simulink model "rob_dynModel"  (R2022b)
settings: Solver=VariableStepAuto  StartTime=0.0  StopTime=100  RelTol=1e-3
values from neighbouring files (symbols this model uses):
  B1 = 2    [inputConstants.m]    (also in inputContants.mat)
  B2 = 2    [inputConstants.m]    (also in inputContants.mat)
  g = 9.81    [inputConstants.m]    (also in inputContants.mat)
  l1 = 0.75    [inputConstants.m]    (also in inputContants.mat)
  l2 = 0.75    [inputConstants.m]    (also in inputContants.mat)
  m1 = 10    [inputConstants.m]    (also in inputContants.mat)
  m2 = 10    [inputConstants.m]    (also in inputContants.mat)
undefined symbols (not defined in the file or in its folder): sigbuilder_block
libraries: simulink_extras x4, slpidlib x2
settings Model: Creator=Marek Sýkorka  LastModifiedBy=Marek Sýkorka

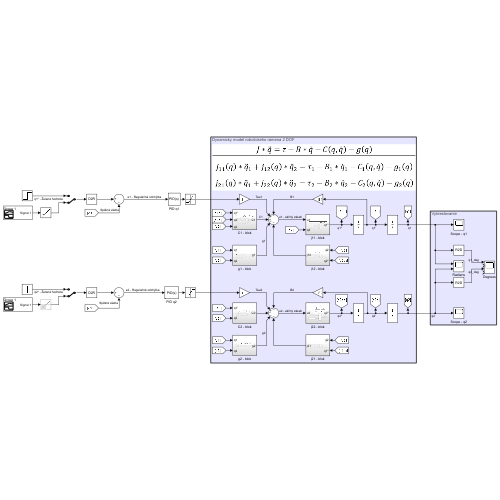
[thumbnail: Simulink's stored preview of the top-level diagram]
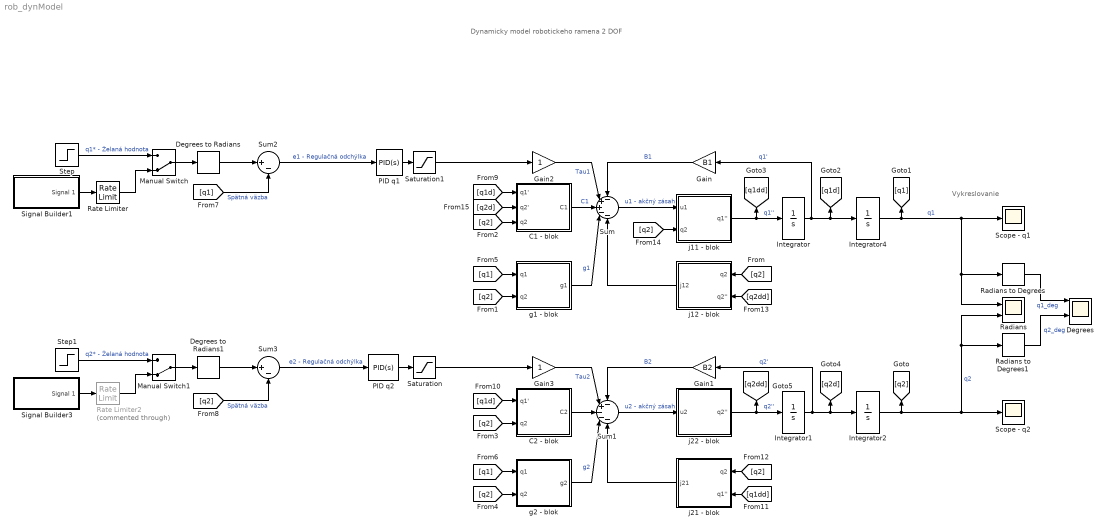
== system rob_dynModel ==
  note: Vykreslovanie
  note: Dynamicky model robotickeho ramena 2 DOF
  C1 - blok : Subsystem
  C2 - blok : Subsystem
  Degrees : Scope  NumInputPorts=4
  Degrees to Radians : simulink_extras/Transformations/Degrees to Radians
  Degrees to Radians1 : simulink_extras/Transformations/Degrees to Radians
  Gain : Gain  Gain=B1
  Gain1 : Gain  Gain=B2
  Gain2 : Gain
  Gain3 : Gain
  Integrator{,1..2,4} (4 alike) : Integrator
  Manual Switch : ManualSwitch  CurrentSetting=0
  Manual Switch1 : ManualSwitch  CurrentSetting=0
  PID q1 : slpidlib/PID Controller  Controller=PID  Form=Parallel  TimeDomain=Continuous-time  UseExternalTs=off  SampleTime=-1  IntegratorMethod=Forward Euler  FilterMethod=Forward Euler  ControllerParametersSource=internal  P=15000  I=6500  UseKiTs=off  D=6000  N=1000  UseFilter=on  TunerSelectOption=Transfer Function Based (PID Tuner App)  ZeroCross=off  InitialConditionSource=internal  InitialConditionForIntegrator=0  InitialConditionForFilter=0  DifferentiatorICPrevScaledInput=0  ExternalReset=none  TrackingMode=off  Kt=1  LimitOutput=off  SatLimitsSource=internal  UpperSaturationLimit=inf  LowerSaturationLimit=-inf  LinearizeAsGain=on  AntiWindupMode=none  Kb=1  LimitIntegrator=off  UpperIntegratorSaturationLimit=inf  LowerIntegratorSaturationLimit=-inf  POutMin=[]  POutMax=[]  IOutMin=[]  IOutMax=[]  DOutMin=[]  DOutMax=[]  NOutMin=[]  NOutMax=[]  SumOutMin=[]  SumOutMax=[]  SaturationOutMin=[]  SaturationOutMax=[]  PParamMin=[]  PParamMax=[]  IParamMin=[]  IParamMax=[]  DParamMin=[]  DParamMax=[]  NParamMin=[]  NParamMax=[]  KbParamMin=[]  KbParamMax=[]  KtParamMin=[]  KtParamMax=[]  KbOutMin=[]  KbOutMax=[]  KtOutMin=[]  KtOutMax=[]  IntegratorOutMin=[]  IntegratorOutMax=[]  FilterOutMin=[]  FilterOutMax=[]  SumI1OutMin=[]  SumI1OutMax=[]  SumI2OutMin=[]  SumI2OutMax=[]  SumI3OutMin=[]  SumI3OutMax=[]  SumI4OutMin=[]  SumI4OutMax=[]  SumDOutMin=[]  SumDOutMax=[]  DifferentiatorOutMin=[]  DifferentiatorOutMax=[]  FilterDiffOutCoefMin=[]  FilterDiffOutCoefMax=[]  ReciprocalOutMin=[]  ReciprocalOutMax=[]  SumDenOutMin=[]  SumDenOutMax=[]  SumNumOutMin=[]  SumNumOutMax=[]  DivideOutMin=[]  DivideOutMax=[]  UdiffTsProdOutMin=[]  UdiffTsProdOutMax=[]  NTsProdOutMin=[]  NTsProdOutMax=[]  UintegralTsProdOutMin=[]  UintegralTsProdOutMax=[]  UngainTsProdOutMin=[]  UngainTsProdOutMax=[]  ClampingZeroOutDataTypeStr=Inherit: Inherit via back propagation  ClampingZeroOutMin=[]  ClampingZeroOutMax=[]  FilterDenConstantOutDataTypeStr=Inherit: Inherit via back propagation  FilterDenConstantOutMin=[]  FilterDenConstantOutMax=[]  PCopyOutDataTypeStr=Inherit: Inherit via back propagation  PCopyOutMin=[]  PCopyOutMax=[]  NCopyOutDataTypeStr=Inherit: Inherit via back propagation  NCopyOutMin=[]  NCopyOutMax=[]  IntegratorContinuousStateAttributes=''  IntegratorStateMustResolveToSignalObject=off  IntegratorRTWStateStorageClass=Auto  FilterContinuousStateAttributes=''  FilterStateMustResolveToSignalObject=off  FilterRTWStateStorageClass=Auto  ParallelPVariant=InternalParameters  IdealPVariant=Disabled  IVariant=InternalParameters  DVariant=InternalParameters  IntegratorVariant=Continuous  SatVariant=Disabled  AWVariant=Passthrough  PCopyVariant=Disabled  TRVariant=Disabled  FdbkBlocksVariant=Forward  IdealPFdbkVariant=Disabled  SatFdbkVariant=Disabled  DerivativeFilterVariant=ContFilter  NVariant=InternalParameters  NCopyVariant=Disabled  FilterICVariant=InternalICsFilter  IntegratorICVariant=InternalICs  ExternalResetVariant=Disabled  TRSumVariant=Passthrough  SumFdbkVariant=Disabled  SumVariant=Sum_PID  TsampFilterVariant=InternalTs  TsampNgainVariant=Passthrough  TsampIntegralVariant=Passthrough  ExternalSaturationOutDataTypeStr=Inherit: Same as second input
  PID q2 : slpidlib/PID Controller  Controller=PID  Form=Parallel  TimeDomain=Continuous-time  UseExternalTs=off  SampleTime=-1  IntegratorMethod=Forward Euler  FilterMethod=Forward Euler  ControllerParametersSource=internal  P=10000  I=5000  UseKiTs=off  D=4000  N=350  UseFilter=on  TunerSelectOption=Transfer Function Based (PID Tuner App)  InitialConditionSource=internal  InitialConditionForIntegrator=0  InitialConditionForFilter=0  DifferentiatorICPrevScaledInput=0  ExternalReset=none  TrackingMode=off  Kt=1  LimitOutput=off  SatLimitsSource=internal  UpperSaturationLimit=inf  LowerSaturationLimit=-inf  LinearizeAsGain=on  AntiWindupMode=none  Kb=1  LimitIntegrator=off  UpperIntegratorSaturationLimit=inf  LowerIntegratorSaturationLimit=-inf  POutMin=[]  POutMax=[]  IOutMin=[]  IOutMax=[]  DOutMin=[]  DOutMax=[]  NOutMin=[]  NOutMax=[]  SumOutMin=[]  SumOutMax=[]  SaturationOutMin=[]  SaturationOutMax=[]  PParamMin=[]  PParamMax=[]  IParamMin=[]  IParamMax=[]  DParamMin=[]  DParamMax=[]  NParamMin=[]  NParamMax=[]  KbParamMin=[]  KbParamMax=[]  KtParamMin=[]  KtParamMax=[]  KbOutMin=[]  KbOutMax=[]  KtOutMin=[]  KtOutMax=[]  IntegratorOutMin=[]  IntegratorOutMax=[]  FilterOutMin=[]  FilterOutMax=[]  SumI1OutMin=[]  SumI1OutMax=[]  SumI2OutMin=[]  SumI2OutMax=[]  SumI3OutMin=[]  SumI3OutMax=[]  SumI4OutMin=[]  SumI4OutMax=[]  SumDOutMin=[]  SumDOutMax=[]  DifferentiatorOutMin=[]  DifferentiatorOutMax=[]  FilterDiffOutCoefMin=[]  FilterDiffOutCoefMax=[]  ReciprocalOutMin=[]  ReciprocalOutMax=[]  SumDenOutMin=[]  SumDenOutMax=[]  SumNumOutMin=[]  SumNumOutMax=[]  DivideOutMin=[]  DivideOutMax=[]  UdiffTsProdOutMin=[]  UdiffTsProdOutMax=[]  NTsProdOutMin=[]  NTsProdOutMax=[]  UintegralTsProdOutMin=[]  UintegralTsProdOutMax=[]  UngainTsProdOutMin=[]  UngainTsProdOutMax=[]  ClampingZeroOutDataTypeStr=Inherit: Inherit via back propagation  ClampingZeroOutMin=[]  ClampingZeroOutMax=[]  FilterDenConstantOutDataTypeStr=Inherit: Inherit via back propagation  FilterDenConstantOutMin=[]  FilterDenConstantOutMax=[]  PCopyOutDataTypeStr=Inherit: Inherit via back propagation  PCopyOutMin=[]  PCopyOutMax=[]  NCopyOutDataTypeStr=Inherit: Inherit via back propagation  NCopyOutMin=[]  NCopyOutMax=[]  IntegratorContinuousStateAttributes=''  IntegratorStateMustResolveToSignalObject=off  IntegratorRTWStateStorageClass=Auto  FilterContinuousStateAttributes=''  FilterStateMustResolveToSignalObject=off  FilterRTWStateStorageClass=Auto  ParallelPVariant=InternalParameters  IdealPVariant=Disabled  IVariant=InternalParameters  DVariant=InternalParameters  IntegratorVariant=Continuous  SatVariant=Disabled  AWVariant=Passthrough  PCopyVariant=Disabled  TRVariant=Disabled  FdbkBlocksVariant=Forward  IdealPFdbkVariant=Disabled  SatFdbkVariant=Disabled  DerivativeFilterVariant=ContFilter  NVariant=InternalParameters  NCopyVariant=Disabled  FilterICVariant=InternalICsFilter  IntegratorICVariant=InternalICs  ExternalResetVariant=Disabled  TRSumVariant=Passthrough  SumFdbkVariant=Disabled  SumVariant=Sum_PID  TsampFilterVariant=InternalTs  TsampNgainVariant=Passthrough  TsampIntegralVariant=Passthrough  ExternalSaturationOutDataTypeStr=Inherit: Same as second input
  Radians : Scope  NumInputPorts=2
  Radians to Degrees : simulink_extras/Transformations/Radians to Degrees
  Radians to Degrees1 : simulink_extras/Transformations/Radians to Degrees
  Rate Limiter : RateLimiter  RisingSlewLimit=180  FallingSlewLimit=-180
  Rate Limiter2 : RateLimiter  Commented=through  RisingSlewLimit=180  FallingSlewLimit=-180
  Saturation : Saturate  UpperLimit=2000  LowerLimit=-2000
  Saturation1 : Saturate  UpperLimit=2000  LowerLimit=-2000
  Scope - q1 : Scope
  Scope - q2 : Scope
  Signal Builder1 : Subsystem  Tag=STV Subsys  LoadFcn=sigbuilder_block('load');  StartFcn=sigbuilder_block('start');  StopFcn=sigbuilder_block('stop');  ClipboardFcn=sigbuilder_block('clipboard');  mask(Sigbuilder block){tuvar=[0:10]}
      mask help: Simulink:masks:SigbuilderBlock_MD
      mask init:
      | if ~strcmp(get_param(bdroot(gcbh),'SimulationStatus'),'stopped') tuvar = sigbuilder_block('maskInit'); end
      settings: CopyFcn=sigbuilder_block('copy');  DeleteFcn=sigbuilder_block('delete');  ModelCloseFcn=sigbuilder_block('modelClose');  PreSaveFcn=sigbuilder_block('preSave');  PauseFcn=sigbuilder_block('pause');  ContinueFcn=sigbuilder_block('continue');  NameChangeFcn=sigbuilder_block('namechange');  OpenFcn=sigbuilder_block('open',[5.4 0 1141.2 552.6 ]);  CloseFcn=sigbuilder_block('close');
      mask Display: plot(0, 0, 100, 100,[2, 2, 32, 32, 2], [68, 8, 8, 68, 68],[32, 2], [38, 38], [32, 19, 2],[53, 60, 44], [32, 17, 17, 2],[16, 16, 31, 31]);txt = getActiveGroup(gcbh);text(2, 100, txt,'verticalAlignment', 'top');
  Signal Builder3 : Subsystem  Tag=STV Subsys  LoadFcn=sigbuilder_block('load');  StartFcn=sigbuilder_block('start');  StopFcn=sigbuilder_block('stop');  ClipboardFcn=sigbuilder_block('clipboard');  mask(Sigbuilder block){tuvar=[0:10]}
      mask help: Simulink:masks:SigbuilderBlock_MD
      mask init:
      | if ~strcmp(get_param(bdroot(gcbh),'SimulationStatus'),'stopped') tuvar = sigbuilder_block('maskInit'); end
      settings: CopyFcn=sigbuilder_block('copy');  DeleteFcn=sigbuilder_block('delete');  ModelCloseFcn=sigbuilder_block('modelClose');  PreSaveFcn=sigbuilder_block('preSave');  PauseFcn=sigbuilder_block('pause');  ContinueFcn=sigbuilder_block('continue');  NameChangeFcn=sigbuilder_block('namechange');  OpenFcn=sigbuilder_block('open',[5.4 0 1141.2 552.6 ]);  CloseFcn=sigbuilder_block('close');
      mask Display: plot(0, 0, 100, 100,[2, 2, 32, 32, 2], [68, 8, 8, 68, 68],[32, 2], [38, 38], [32, 19, 2],[53, 60, 44], [32, 17, 17, 2],[16, 16, 31, 31]);txt = getActiveGroup(gcbh);text(2, 100, txt,'verticalAlignment', 'top');
  Step : Step  Time=0  After=90  SampleTime=0
  Step1 : Step  Time=0  After=90  SampleTime=0
  Sum : Sum  Inputs=-++--
  Sum1 : Sum  Inputs=-+---
  Sum2 : Sum  Inputs=|+-
  Sum3 : Sum  Inputs=|+-
  g1 - blok : Subsystem
  g2 - blok : Subsystem
  j11 - blok : Subsystem
  j12 - blok : Subsystem
  j21 - blok : Subsystem
  j22 - blok : Subsystem
  wires:
  Integrator/1 -> Gain/1, Integrator4/1, [q1d]  "q1'"
  Integrator4/1 -> Scope - q1/1, Radians to Degrees/1, Radians/1, [q1]  "q1"
  Gain/1 -> Sum/1  "B1"
  Integrator2/1 -> Radians to Degrees1/1, Radians/2, Scope - q2/1, [q2]  "q2"
  j22 - blok/1(q2'') -> [q2dd], Integrator1/1  "q2''"
  Integrator1/1 -> [q2d], Integrator2/1, Gain1/1  "q2'"
  C1 - blok/1(C1) -> Sum/3  "C1"
  g1 - blok/1(g1) -> Sum/4  "g1"
  Sum/1 -> j11 - blok/1(u1)  "u1 - akčný zásah"
  j11 - blok/1(q1'') -> Integrator/1, [q1dd]  "q1''"
  j12 - blok/1(j12) -> Sum/5
  j21 - blok/1(j21) -> Sum1/5
  g2 - blok/1(g2) -> Sum1/4  "g2"
  C2 - blok/1(C2) -> Sum1/3
  Gain1/1 -> Sum1/1  "B2"
  Sum1/1 -> j22 - blok/1(u2)  "u2 - akčný zásah"
  Radians to Degrees/1 -> Degrees/1  "q1_deg"
  Radians to Degrees1/1 -> Degrees/3  "q2_deg"
  [q2] -> j12 - blok/1(q2)
  [q2] -> C1 - blok/3(q2)
  [q2] -> g1 - blok/2(q2)
  [q2] -> C2 - blok/2(q2)
  [q2] -> g2 - blok/2(q2)
  [q1] -> g1 - blok/1(q1)
  [q1] -> g2 - blok/1(q1)
  [q1] -> Sum2/2  "Spätná väzba"
  [q2] -> Sum3/2  "Spätná väzba"
  [q1d] -> C1 - blok/1(q1')
  [q1d] -> C2 - blok/1(q1')
  [q2dd] -> j12 - blok/2(q2'')
  [q2] -> j11 - blok/2(q2)
  [q2d] -> C1 - blok/2(q2')
  PID q2/1 -> Saturation/1
  Sum2/1 -> PID q1/1  "e1 - Regulačná odchýlka"
  Gain2/1 -> Sum/2  "Tau1"
  [q2] -> j21 - blok/1(q2)
  [q1dd] -> j21 - blok/2(q1'')
  Gain3/1 -> Sum1/2  "Tau2"
  Sum3/1 -> PID q2/1  "e2 - Regulačná odchýlka"
  PID q1/1 -> Saturation1/1
  Degrees to Radians/1 -> Sum2/1
  Degrees to Radians1/1 -> Sum3/1
  Manual Switch/1 -> Degrees to Radians/1
  Step/1 -> Manual Switch/1  "q1* - Želaná hodnota"
  Signal Builder1/1(Signal 1) -> Rate Limiter/1
  Step1/1 -> Manual Switch1/1  "q2* - Želaná hodnota"
  Signal Builder3/1(Signal 1) -> Rate Limiter2/1
  Manual Switch1/1 -> Degrees to Radians1/1
  Rate Limiter2/1 -> Manual Switch1/2
  Rate Limiter/1 -> Manual Switch/2
  Saturation/1 -> Gain3/1
  Saturation1/1 -> Gain2/1

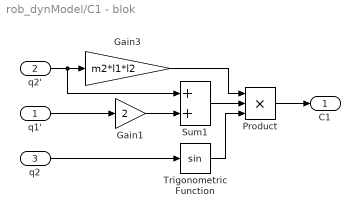
== system rob_dynModel/C1 - blok ==
  q1' : Inport
  q2' : Inport  Port=2
  q2 : Inport  Port=3
  Gain1 : Gain  Gain=2
  Gain3 : Gain  Gain=m2*l1*l2
  Product : Product  Inputs=3
  Sum1 : Sum
  Trigonometric Function : Trigonometry
  C1 : Outport
  wires:
  Gain3/1 -> Product/1
  q2'/1 -> Gain3/1, Sum1/1
  Sum1/1 -> Product/2
  q2/1 -> Trigonometric Function/1
  Gain1/1 -> Sum1/2
  q1'/1 -> Gain1/1
  Trigonometric Function/1 -> Product/3
  Product/1 -> C1/1

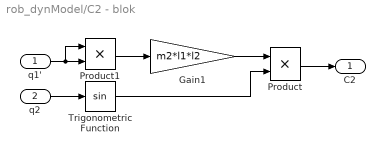
== system rob_dynModel/C2 - blok ==
  q1' : Inport
  q2 : Inport  Port=2
  Gain1 : Gain  Gain=m2*l1*l2
  Product : Product
  Product1 : Product
  Trigonometric Function : Trigonometry
  C2 : Outport
  wires:
  q2/1 -> Trigonometric Function/1
  q1'/1 -> Product1/1, Product1/2
  Product/1 -> C2/1
  Gain1/1 -> Product/1
  Product1/1 -> Gain1/1
  Trigonometric Function/1 -> Product/2

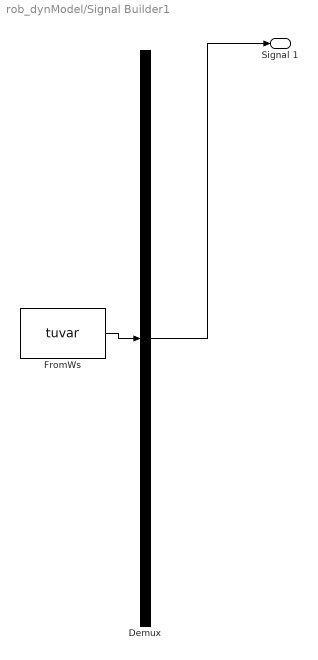
== system rob_dynModel/Signal Builder1 ==
  Demux : Demux  Tag=STV Demux  Outputs=1
      settings: DisplayOption=none
  FromWs : FromWorkspace  Tag=STV FromWs  VariableName=tuvar
      SigBuilderData=|
      | common.afterFinalStr = 'Extrapolate'
      | common.sampleTime = 0
      | dataSet.timeRange = [0 100]
      | dataSet.name = 'Group 1'
      | sbobj.Groups.Name = 'Group 1'
      | sbobj.Groups.Signals.Name = 'Signal 1'
      | sbobj.Groups.Signals.XData = [0 1 1.5 1.5 10 10 10.5 19.5 20 29.5 30 100]
      | sbobj.Groups.Signals.YData = [0 0 90 90 90 90 120 120 45 45 0 0]
      | sbobj.Groups.TimeRange = [0 100]
  Signal 1 : Outport  Tag=STV Outport
  wires:
  FromWs/1 -> Demux/1
  Demux/1 -> Signal 1/1

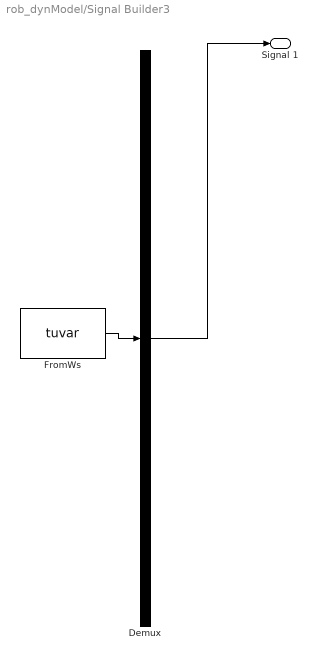
== system rob_dynModel/Signal Builder3 ==
  Demux : Demux  Tag=STV Demux  Outputs=1
      settings: DisplayOption=none
  FromWs : FromWorkspace  Tag=STV FromWs  VariableName=tuvar
      SigBuilderData=|
      | common.afterFinalStr = 'Extrapolate'
      | common.sampleTime = 0
      | dataSet.timeRange = [0 100]
      | dataSet.name = 'Group 1'
      | sbobj.Groups.Name = 'Group 1'
      | sbobj.Groups.Signals.Name = 'Signal 1'
      | sbobj.Groups.Signals.XData = [0 10 10.5 20 20.5 29.5 30 39.5 40 100]
      | sbobj.Groups.Signals.YData = [0 0 90 90 120 120 45 45 0 0]
      | sbobj.Groups.TimeRange = [0 100]
  Signal 1 : Outport  Tag=STV Outport
  wires:
  FromWs/1 -> Demux/1
  Demux/1 -> Signal 1/1

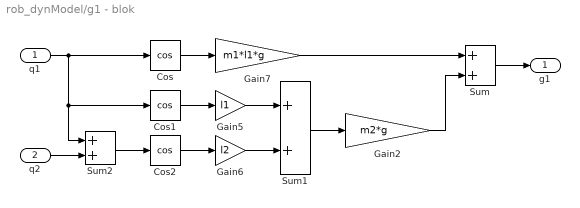
== system rob_dynModel/g1 - blok ==
  q1 : Inport
  q2 : Inport  Port=2
  Cos : Trigonometry  Operator=cos
  Cos1 : Trigonometry  Operator=cos
  Cos2 : Trigonometry  Operator=cos
  Gain2 : Gain  Gain=m2*g
  Gain5 : Gain  Gain=l1
  Gain6 : Gain  Gain=l2
  Gain7 : Gain  Gain=m1*l1*g
  Sum : Sum
  Sum1 : Sum
  Sum2 : Sum
  g1 : Outport
  wires:
  q1/1 -> Cos/1, Sum2/1, Cos1/1
  Gain7/1 -> Sum/1
  q2/1 -> Sum2/2
  Sum2/1 -> Cos2/1
  Cos1/1 -> Gain5/1
  Cos2/1 -> Gain6/1
  Gain5/1 -> Sum1/1
  Gain6/1 -> Sum1/2
  Sum/1 -> g1/1
  Cos/1 -> Gain7/1
  Sum1/1 -> Gain2/1
  Gain2/1 -> Sum/2

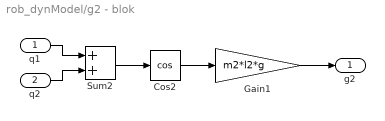
== system rob_dynModel/g2 - blok ==
  q1 : Inport
  q2 : Inport  Port=2
  Cos2 : Trigonometry  Operator=cos
  Gain1 : Gain  Gain=m2*l2*g
  Sum2 : Sum
  g2 : Outport
  wires:
  Sum2/1 -> Cos2/1
  q1/1 -> Sum2/1
  Gain1/1 -> g2/1
  Cos2/1 -> Gain1/1
  q2/1 -> Sum2/2

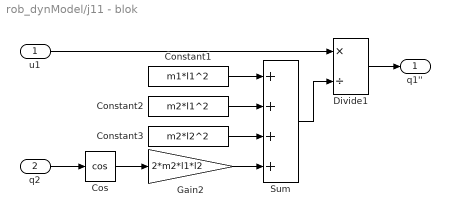
== system rob_dynModel/j11 - blok ==
  u1 : Inport
  q2 : Inport  Port=2
  Constant1 : Constant  Value=m1*l1^2
  Constant2 : Constant  Value=m2*l1^2
  Constant3 : Constant  Value=m2*l2^2
  Cos : Trigonometry  Operator=cos
  Divide1 : Product  Inputs=*/
  Gain2 : Gain  Gain=2*m2*l1*l2
  Sum : Sum  Inputs=++++
  q1'' : Outport
  wires:
  Gain2/1 -> Sum/4
  Cos/1 -> Gain2/1
  q2/1 -> Cos/1
  Constant2/1 -> Sum/2
  u1/1 -> Divide1/1
  Constant1/1 -> Sum/1
  Constant3/1 -> Sum/3
  Sum/1 -> Divide1/2
  Divide1/1 -> q1''/1

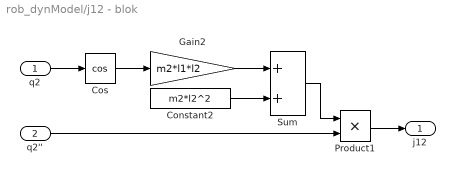
== system rob_dynModel/j12 - blok ==
  q2 : Inport
  q2'' : Inport  Port=2
  Constant2 : Constant  Value=m2*l2^2
  Cos : Trigonometry  Operator=cos
  Gain2 : Gain  Gain=m2*l1*l2
  Product1 : Product
  Sum : Sum
  j12 : Outport
  wires:
  q2/1 -> Cos/1
  Product1/1 -> j12/1
  Cos/1 -> Gain2/1
  q2''/1 -> Product1/2
  Sum/1 -> Product1/1
  Gain2/1 -> Sum/1
  Constant2/1 -> Sum/2

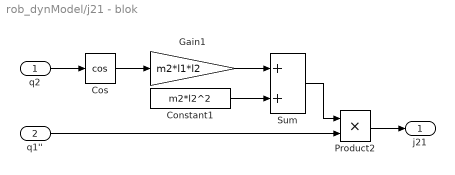
== system rob_dynModel/j21 - blok ==
  q2 : Inport
  q1'' : Inport  Port=2
  Constant1 : Constant  Value=m2*l2^2
  Cos : Trigonometry  Operator=cos
  Gain1 : Gain  Gain=m2*l1*l2
  Product2 : Product
  Sum : Sum
  j21 : Outport
  wires:
  Cos/1 -> Gain1/1
  q2/1 -> Cos/1
  Gain1/1 -> Sum/1
  Constant1/1 -> Sum/2
  Product2/1 -> j21/1
  q1''/1 -> Product2/2
  Sum/1 -> Product2/1

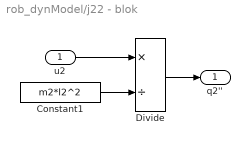
== system rob_dynModel/j22 - blok ==
  u2 : Inport
  Constant1 : Constant  Value=m2*l2^2
  Divide : Product  Inputs=*/
  q2'' : Outport
  wires:
  Constant1/1 -> Divide/2
  u2/1 -> Divide/1
  Divide/1 -> q2''/1
